simulink model "CM4_ADC_Test"  (R2020b)
settings: Solver=FixedStepAuto  StartTime=0.0  StopTime=60  FixedStep=0.01  RelTol=1e-3  EnableMultiTasking=on
libraries: simulink x2, embdlinuxlib x2, raspberrypiCommlib x1
settings Model: Creator=cbeal  LastModifiedBy=cbeal
settings SolverCC: PositivePriorityOrder=on
settings DataIOCC: ReturnWorkspaceOutputs=off
settings OptimizationCC: EnhancedBackFolding=on  PassReuseOutputArgsAs=Individual arguments  ZeroExternalMemoryAtStartup=off  ZeroInternalMemoryAtStartup=off  MaxStackSize=64  OptimizeBlockOrder=speed  DifferentSizesBufferReuse=on  OptimizationCustomize=off  EfficientTunableParamExpr=on
settings DebuggingCC: ParameterTunabilityLossMsg=error
settings HardwareCC: ProdBitPerPointer=32  ProdBitPerSizeT=32  ProdBitPerPtrDiffT=32  ProdLargestAtomicInteger=Long  ProdLargestAtomicFloat=Double  ProdWordSize=32  ProdLongLongMode=on  ProdHWDeviceType=ARM Compatible->ARM Cortex
settings RTWCC: Description=Embedded Coder  SystemTargetFile=ert.tlc  HardwareBoard=Raspberry Pi  TLCOptions="-aInlineSetEventsForThisBaseRateFcn=TLC_FALSE -aSuppressMultiTaskScheduler=TLC_FALSE  -aRateBasedStepFcn=0"  TemplateMakefile=ert_default_tmf  Toolchain=GNU GCC Raspberry Pi  BuildConfiguration=Faster Runs
settings CodeAppCC: ForceParamTrailComments=on  IgnoreCustomStorageClasses=off  OperatorAnnotations=on  SimulinkDataObjDesc=on  SFDataObjDesc=on  InsertBlockDesc=on
settings ERTTargetCC: SupportVariableSizeSignals=on  ExtModeTransport=2  ExtModeMexFile=ext_xcp  ExtModeIntrfLevel=Level2 - Open

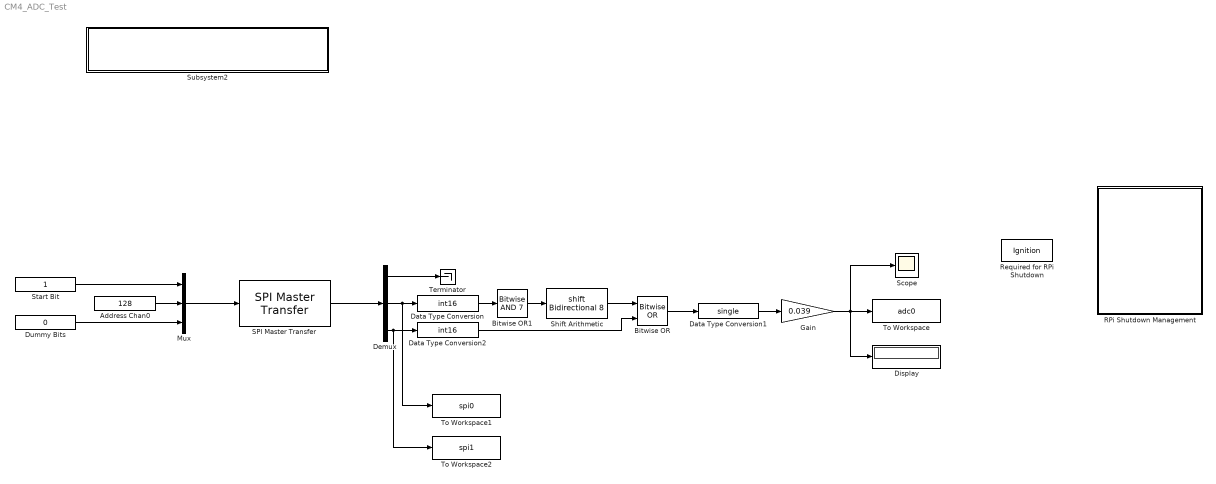
== system CM4_ADC_Test ==
  Address Chan0 : Constant  Value=128
  Bitwise OR : simulink/Logic and Bit Operations/Bitwise Operator  logicop=OR  UseBitMask=off  NumInputPorts=2  BitMask=bin2dec('11011001')  BitMaskRealWorld=Stored Integer
  Bitwise OR1 : simulink/Logic and Bit Operations/Bitwise Operator  logicop=AND  UseBitMask=on  BitMask=7  BitMaskRealWorld=Stored Integer
  Data Type Conversion : DataTypeConversion  OutDataTypeStr=int16  ConvertRealWorld=Stored Integer (SI)
  Data Type Conversion1 : DataTypeConversion  OutDataTypeStr=single
  Data Type Conversion2 : DataTypeConversion  OutDataTypeStr=int16  ConvertRealWorld=Stored Integer (SI)
  Demux : Demux  Outputs=3
  Display : Display
  Dummy Bits : Constant  Value=0
  Gain : Gain  Gain=0.039
  Mux : Mux  Inputs=3
  RPi Shutdown Management : Subsystem
  Required for RPi Shutdown : DataStoreMemory  DataStoreName=Ignition  ReadBeforeWriteMsg=warning  WriteAfterWriteMsg=warning  WriteAfterReadMsg=warning  ShowAdditionalParam=off  OutDataTypeStr=uint8
  SPI Master Transfer : raspberrypiCommlib/SPI Master Transfer  BoardProperty=Pi 4 Model B  SSPin=SPI0_CE1  SPIModule=uint32(0)  Mode=Master  BusSpeed=1000000  Pin=uint32(0)  FirstBitToTransfer=Most significant bit (MSB)  ClockMode=0  BlockFunction=Transfer  RegisterAddress=0  OutputDataType=int8  OutputDataLength=1
      settings: SourceProductBaseCode=RASPPI
  Scope : Scope
  Shift Arithmetic : ArithShift  BitShiftNumber=8
  Start Bit : Constant
  Subsystem2 : Subsystem
      mask Display:
      | scl=1/4;
      | patch(scl*[0,52,90,54],scl*[16,55,146,146],[16/255,118/255,188/255],'bottom-left');
      | patch(scl*[0,27,82,77,68],scl*[16,0,42,62,69],[46/255,49/255,146/255],'bottom-left');
      | patch(scl*[89,125,90,68],scl*[16,16,146,91],[0,0,0],'bottom-left');
      | disp('Run Once at Startup');
  Terminator : Terminator
  To Workspace : ToWorkspace  VariableName=adc0  SampleTime=-1
      settings: Save2DSignal=2-D array (concatenate along first dimension)
  To Workspace1 : ToWorkspace  VariableName=spi0  SampleTime=-1
      settings: Save2DSignal=2-D array (concatenate along first dimension)
  To Workspace2 : ToWorkspace  VariableName=spi1  SampleTime=-1
      settings: Save2DSignal=2-D array (concatenate along first dimension)
  wires:
  Mux/1 -> SPI Master Transfer/1
  Start Bit/1 -> Mux/1
  Address Chan0/1 -> Mux/2
  Dummy Bits/1 -> Mux/3
  SPI Master Transfer/1 -> Demux/1
  Demux/2 -> To Workspace1/1, Data Type Conversion/1
  Demux/1 -> Terminator/1
  Demux/3 -> To Workspace2/1, Data Type Conversion2/1
  Shift Arithmetic/1 -> Bitwise OR/1
  Data Type Conversion2/1 -> Bitwise OR/2
  Bitwise OR/1 -> Data Type Conversion1/1
  Data Type Conversion1/1 -> Gain/1
  Gain/1 -> Display/1, Scope/1, To Workspace/1
  Data Type Conversion/1 -> Bitwise OR1/1
  Bitwise OR1/1 -> Shift Arithmetic/1

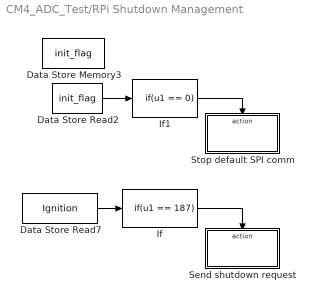
== system CM4_ADC_Test/RPi Shutdown Management ==
  Data Store Memory3 : DataStoreMemory  DataStoreName=init_flag  ReadBeforeWriteMsg=warning  WriteAfterWriteMsg=warning  WriteAfterReadMsg=warning  ShowAdditionalParam=off  OutDataTypeStr=uint8
  Data Store Read2 : DataStoreRead  DataStoreName=init_flag
  Data Store Read7 : DataStoreRead  DataStoreName=Ignition
  If : If  IfExpression=u1 == 187  ShowElse=off
  If1 : If  IfExpression=u1 == 0  ShowElse=off
  Send shutdown request : Subsystem  TreatAsAtomicUnit=on
  Stop default SPI comm : Subsystem  TreatAsAtomicUnit=on
  wires:
  If/1 -> Send shutdown request/Action
  Data Store Read7/1 -> If/1
  If1/1 -> Stop default SPI comm/Action
  Data Store Read2/1 -> If1/1

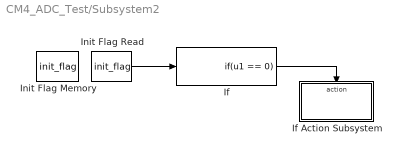
== system CM4_ADC_Test/Subsystem2 ==
  If : If  IfExpression=u1 == 0  ShowElse=off
  If Action Subsystem : Subsystem  TreatAsAtomicUnit=on
  Init Flag Memory : DataStoreMemory  DataStoreName=init_flag  ReadBeforeWriteMsg=warning  WriteAfterWriteMsg=warning  WriteAfterReadMsg=warning  ShowAdditionalParam=off  OutDataTypeStr=uint32
  Init Flag Read : DataStoreRead  DataStoreName=init_flag
  wires:
  Init Flag Read/1 -> If/1
  If/1 -> If Action Subsystem/Action

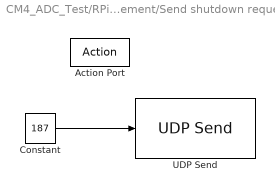
== system CM4_ADC_Test/RPi Shutdown Management/Send shutdown request ==
  Action Port : ActionPort  ActionPortLabel=if(u1 == 187)
  Constant : Constant  Value=187  OutDataTypeStr=uint8
  UDP Send : embdlinuxlib/UDP Send  remoteURL='127.0.0.1'  remotePort=5005  localURL='255.255.255.255'  localPortSource=Automatically determine  localPort=-1  sampletime=-1  blockPlatform=Raspberry Pi  separateLengthPort=0
      settings: SourceProductBaseCode=SC_BEAGLEBONE_BLUE,NVIDIA,RASPPI
  wires:
  Constant/1 -> UDP Send/1

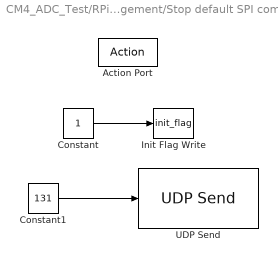
== system CM4_ADC_Test/RPi Shutdown Management/Stop default SPI comm ==
  Action Port : ActionPort  ActionPortLabel=if(u1 == 0)
  Constant : Constant  OutDataTypeStr=uint8
  Constant1 : Constant  Value=131  OutDataTypeStr=uint8
  Init Flag Write : DataStoreWrite  DataStoreName=init_flag
  UDP Send : embdlinuxlib/UDP Send  remoteURL='127.0.0.1'  remotePort=5005  localURL='255.255.255.255'  localPortSource=Automatically determine  localPort=-1  sampletime=-1  blockPlatform=Raspberry Pi  separateLengthPort=0
      settings: SourceProductBaseCode=SC_BEAGLEBONE_BLUE,NVIDIA,RASPPI
  wires:
  Constant/1 -> Init Flag Write/1
  Constant1/1 -> UDP Send/1

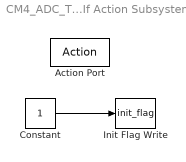
== system CM4_ADC_Test/Subsystem2/If Action Subsystem ==
  Action Port : ActionPort  ActionPortLabel=if(u1 == 0)
  Constant : Constant  OutDataTypeStr=uint32
  Init Flag Write : DataStoreWrite  DataStoreName=init_flag
  wires:
  Constant/1 -> Init Flag Write/1
